simulink model "Battery_Model"  (R2019b)
settings: configuration reference "BMS_Sw_CodeGenConfig" (kept outside this file)
undefined symbols (not defined in the file): Battery, TempInit, ts
libraries: fl_lib x2765, nesl_utility x1565, ee_lib x384, simulink x384, BatteryPack_lib x3
(part 23 of 33)

== system Battery_Model/Battery_Pack/Battery_Pack_7Modules/Cell_3p05/Cell_Module_1 ==
  AmbientTemp : Inport
  Battery_Cell001 : ee_lib/Sources/Battery (Table-Based)  SOC_vec=Battery.SOC_LUT  T_dependence=ee.enum.temperature_dependence.yes  T_vec=Battery.Temperature_LUT K  V0_mat=Battery.Em_LUT V  V0_vec=[3.1, 3.27, 3.31, 3.5] V  R0_mat=Battery.R0_LUT Ohm  R0_vec=[.015, .017, .012, .013] Ohm  AH_vec=Battery.Capacity_LUT hr*A  AH=4.1 hr*A  prm_leak=ee.enum.battery.prm_leak.disabled  Rleak_vec=[8000, 7000, 6000] Ohm  Rleak=7e3 Ohm  prm_dyn=ee.enum.battery.prm_dyn.rc1  R1_mat=Battery.R1_LUT Ohm  R1_vec=[.076, .022, .007, .043] Ohm  tau1_mat=Battery.R1_LUT.*Battery.C1_LUT s  tau1_vec=[148, 110, 27, 22] s  R2_mat=[.014, .382, .407; .028, .006, .007; .014, .007, .006; .333, .956, .912] Ohm  R2_vec=[.382, .006, .007, .956] Ohm  tau2_mat=[1, 44, 5644; 11, 24, 506; 2, 14, 330; 3310, 13419, 30216] s  tau2_vec=[44, 24, 14, 13419] s  R3_mat=[.014, .382, .407; .028, .006, .007; .014, .007, .006; .333, .956, .912] Ohm  R3_vec=[.382, .006, .007, .956] Ohm  tau3_mat=[1, 44, 5644; 11, 24, 506; 2, 14, 330; 3310, 13419, 30216] s  tau3_vec=[44, 24, 14, 13419] s  R4_mat=[.014, .382, .407; .028, .006, .007; .014, .007, .006; .333, .956, .912] Ohm  R4_vec=[.382, .006, .007, .956] Ohm  tau4_mat=[1, 44, 5644; 11, 24, 506; 2, 14, 330; 3310, 13419, 30216] s  tau4_vec=[44, 24, 14, 13419] s  R5_mat=[.014, .382, .407; .028, .006, .007; .014, .007, .006; .333, .956, .912] Ohm  R5_vec=[.382, .006, .007, .956] Ohm  tau5_mat=[1, 44, 5644; 11, 24, 506; 2, 14, 330; 3310, 13419, 30216] s  tau5_vec=[44, 24, 14, 13419] s  prm_fade=ee.enum.battery.prm_fade.equations  N0=100  dV0=0  dR0=0  dAH=0  dRleak=0  dR1=0  dR2=0  dR3=0  dR4=0  dR5=0  N0vec=[100, 200, 300]  Tfadevec=[298.15, 323.15] K  dV0vec=[0, 0, 0]  dR0vec=[0, 0, 0]  dAHvec=[0, 0, 0]  dRleakvec=[0, 0, 0]  dR1vec=[0, 0, 0]  dR2vec=[0, 0, 0]  dR3vec=[0, 0, 0]  dR4vec=[0, 0, 0]  dR5vec=[0, 0, 0]  dV0mat=[0, 0; 0, 0; 0, 0]  dR0mat=[0, 0; 0, 0; 0, 0]  dAHmat=[0, 0; 0, 0; 0, 0]  dRleakmat=[0, 0; 0, 0; 0, 0]  dR1mat=[0, 0; 0, 0; 0, 0]  dR2mat=[0, 0; 0, 0; 0, 0]  dR3mat=[0, 0; 0, 0; 0, 0]  dR4mat=[0, 0; 0, 0; 0, 0]  dR5mat=[0, 0; 0, 0; 0, 0]  temperature=Battery.TempInit K  i_specify=off  i_priority=None  i=0 A  i_nominal_specify=off  i_nominal_unit=A  i_nominal_value=1  v_specify=off  v_priority=None  v=0 V  v_nominal_specify=off  v_nominal_unit=V  v_nominal_value=1  stateOfCharge_specify=on  stateOfCharge_priority=High  stateOfCharge=(Battery.Capacity_LUT(1) - Battery.Qe_init)/Battery.Capacity_LUT(1)  stateOfCharge_nominal_specify=off  stateOfCharge_nominal_unit=1  stateOfCharge_nominal_value=1  num_cycles_specify=off  num_cycles_priority=High  num_cycles=0  num_cycles_nominal_specify=off  num_cycles_nominal_unit=1  num_cycles_nominal_value=1  thermal_mass=Battery.cell_mass*Battery.cell_Cp_heat J/K  temperature_specify=on  temperature_priority=High  temperature_nominal_specify=off  temperature_nominal_unit=K  temperature_nominal_value=1
      settings: SourceProductName=Simscape Electrical  SourceProductBaseCode=PS  InternalSimscapePortConfiguration="{\"Bottom\":[],\"Left\":[{\"id\":\"p\",\"label\":\"+\",\"type\":\"foundation.electrical.electrical\"},{\"id\":\"soc\",\"label\":\"SOC\",\"type\":\"output\"}],\"Right\":[{\"id\":\"n\",\"label\":\"-\",\"type\":\"foundation.electrical.electrical\"},{\"id\":\"H\",\"label\":\"H\",\"type\":\"foundation.thermal.thermal\"}],\"Top\":[]}"
  Battery_Cell002 : ee_lib/Sources/Battery (Table-Based)  SOC_vec=Battery.SOC_LUT  T_dependence=ee.enum.temperature_dependence.yes  T_vec=Battery.Temperature_LUT K  V0_mat=Battery.Em_LUT V  V0_vec=[3.1, 3.27, 3.31, 3.5] V  R0_mat=Battery.R0_LUT Ohm  R0_vec=[.015, .017, .012, .013] Ohm  AH_vec=Battery.Capacity_LUT hr*A  AH=4.1 hr*A  prm_leak=ee.enum.battery.prm_leak.disabled  Rleak_vec=[8000, 7000, 6000] Ohm  Rleak=7e3 Ohm  prm_dyn=ee.enum.battery.prm_dyn.rc1  R1_mat=Battery.R1_LUT Ohm  R1_vec=[.076, .022, .007, .043] Ohm  tau1_mat=Battery.R1_LUT.*Battery.C1_LUT s  tau1_vec=[148, 110, 27, 22] s  R2_mat=[.014, .382, .407; .028, .006, .007; .014, .007, .006; .333, .956, .912] Ohm  R2_vec=[.382, .006, .007, .956] Ohm  tau2_mat=[1, 44, 5644; 11, 24, 506; 2, 14, 330; 3310, 13419, 30216] s  tau2_vec=[44, 24, 14, 13419] s  R3_mat=[.014, .382, .407; .028, .006, .007; .014, .007, .006; .333, .956, .912] Ohm  R3_vec=[.382, .006, .007, .956] Ohm  tau3_mat=[1, 44, 5644; 11, 24, 506; 2, 14, 330; 3310, 13419, 30216] s  tau3_vec=[44, 24, 14, 13419] s  R4_mat=[.014, .382, .407; .028, .006, .007; .014, .007, .006; .333, .956, .912] Ohm  R4_vec=[.382, .006, .007, .956] Ohm  tau4_mat=[1, 44, 5644; 11, 24, 506; 2, 14, 330; 3310, 13419, 30216] s  tau4_vec=[44, 24, 14, 13419] s  R5_mat=[.014, .382, .407; .028, .006, .007; .014, .007, .006; .333, .956, .912] Ohm  R5_vec=[.382, .006, .007, .956] Ohm  tau5_mat=[1, 44, 5644; 11, 24, 506; 2, 14, 330; 3310, 13419, 30216] s  tau5_vec=[44, 24, 14, 13419] s  prm_fade=ee.enum.battery.prm_fade.equations  N0=100  dV0=0  dR0=0  dAH=0  dRleak=0  dR1=0  dR2=0  dR3=0  dR4=0  dR5=0  N0vec=[100, 200, 300]  Tfadevec=[298.15, 323.15] K  dV0vec=[0, 0, 0]  dR0vec=[0, 0, 0]  dAHvec=[0, 0, 0]  dRleakvec=[0, 0, 0]  dR1vec=[0, 0, 0]  dR2vec=[0, 0, 0]  dR3vec=[0, 0, 0]  dR4vec=[0, 0, 0]  dR5vec=[0, 0, 0]  dV0mat=[0, 0; 0, 0; 0, 0]  dR0mat=[0, 0; 0, 0; 0, 0]  dAHmat=[0, 0; 0, 0; 0, 0]  dRleakmat=[0, 0; 0, 0; 0, 0]  dR1mat=[0, 0; 0, 0; 0, 0]  dR2mat=[0, 0; 0, 0; 0, 0]  dR3mat=[0, 0; 0, 0; 0, 0]  dR4mat=[0, 0; 0, 0; 0, 0]  dR5mat=[0, 0; 0, 0; 0, 0]  temperature=Battery.TempInit K  i_specify=off  i_priority=None  i=0 A  i_nominal_specify=off  i_nominal_unit=A  i_nominal_value=1  v_specify=off  v_priority=None  v=0 V  v_nominal_specify=off  v_nominal_unit=V  v_nominal_value=1  stateOfCharge_specify=on  stateOfCharge_priority=High  stateOfCharge=(Battery.Capacity_LUT(1) - Battery.Qe_init)/Battery.Capacity_LUT(1)  stateOfCharge_nominal_specify=off  stateOfCharge_nominal_unit=1  stateOfCharge_nominal_value=1  num_cycles_specify=off  num_cycles_priority=High  num_cycles=0  num_cycles_nominal_specify=off  num_cycles_nominal_unit=1  num_cycles_nominal_value=1  thermal_mass=Battery.cell_mass*Battery.cell_Cp_heat J/K  temperature_specify=on  temperature_priority=High  temperature_nominal_specify=off  temperature_nominal_unit=K  temperature_nominal_value=1
      settings: SourceProductName=Simscape Electrical  SourceProductBaseCode=PS  InternalSimscapePortConfiguration="{\"Bottom\":[],\"Left\":[{\"id\":\"p\",\"label\":\"+\",\"type\":\"foundation.electrical.electrical\"},{\"id\":\"soc\",\"label\":\"SOC\",\"type\":\"output\"}],\"Right\":[{\"id\":\"n\",\"label\":\"-\",\"type\":\"foundation.electrical.electrical\"},{\"id\":\"H\",\"label\":\"H\",\"type\":\"foundation.thermal.thermal\"}],\"Top\":[]}"
  Battery_Cell003 : ee_lib/Sources/Battery (Table-Based)  SOC_vec=Battery.SOC_LUT  T_dependence=ee.enum.temperature_dependence.yes  T_vec=Battery.Temperature_LUT K  V0_mat=Battery.Em_LUT V  V0_vec=[3.1, 3.27, 3.31, 3.5] V  R0_mat=Battery.R0_LUT Ohm  R0_vec=[.015, .017, .012, .013] Ohm  AH_vec=Battery.Capacity_LUT hr*A  AH=4.1 hr*A  prm_leak=ee.enum.battery.prm_leak.disabled  Rleak_vec=[8000, 7000, 6000] Ohm  Rleak=7e3 Ohm  prm_dyn=ee.enum.battery.prm_dyn.rc1  R1_mat=Battery.R1_LUT Ohm  R1_vec=[.076, .022, .007, .043] Ohm  tau1_mat=Battery.R1_LUT.*Battery.C1_LUT s  tau1_vec=[148, 110, 27, 22] s  R2_mat=[.014, .382, .407; .028, .006, .007; .014, .007, .006; .333, .956, .912] Ohm  R2_vec=[.382, .006, .007, .956] Ohm  tau2_mat=[1, 44, 5644; 11, 24, 506; 2, 14, 330; 3310, 13419, 30216] s  tau2_vec=[44, 24, 14, 13419] s  R3_mat=[.014, .382, .407; .028, .006, .007; .014, .007, .006; .333, .956, .912] Ohm  R3_vec=[.382, .006, .007, .956] Ohm  tau3_mat=[1, 44, 5644; 11, 24, 506; 2, 14, 330; 3310, 13419, 30216] s  tau3_vec=[44, 24, 14, 13419] s  R4_mat=[.014, .382, .407; .028, .006, .007; .014, .007, .006; .333, .956, .912] Ohm  R4_vec=[.382, .006, .007, .956] Ohm  tau4_mat=[1, 44, 5644; 11, 24, 506; 2, 14, 330; 3310, 13419, 30216] s  tau4_vec=[44, 24, 14, 13419] s  R5_mat=[.014, .382, .407; .028, .006, .007; .014, .007, .006; .333, .956, .912] Ohm  R5_vec=[.382, .006, .007, .956] Ohm  tau5_mat=[1, 44, 5644; 11, 24, 506; 2, 14, 330; 3310, 13419, 30216] s  tau5_vec=[44, 24, 14, 13419] s  prm_fade=ee.enum.battery.prm_fade.equations  N0=100  dV0=0  dR0=0  dAH=0  dRleak=0  dR1=0  dR2=0  dR3=0  dR4=0  dR5=0  N0vec=[100, 200, 300]  Tfadevec=[298.15, 323.15] K  dV0vec=[0, 0, 0]  dR0vec=[0, 0, 0]  dAHvec=[0, 0, 0]  dRleakvec=[0, 0, 0]  dR1vec=[0, 0, 0]  dR2vec=[0, 0, 0]  dR3vec=[0, 0, 0]  dR4vec=[0, 0, 0]  dR5vec=[0, 0, 0]  dV0mat=[0, 0; 0, 0; 0, 0]  dR0mat=[0, 0; 0, 0; 0, 0]  dAHmat=[0, 0; 0, 0; 0, 0]  dRleakmat=[0, 0; 0, 0; 0, 0]  dR1mat=[0, 0; 0, 0; 0, 0]  dR2mat=[0, 0; 0, 0; 0, 0]  dR3mat=[0, 0; 0, 0; 0, 0]  dR4mat=[0, 0; 0, 0; 0, 0]  dR5mat=[0, 0; 0, 0; 0, 0]  temperature=Battery.TempInit K  i_specify=off  i_priority=None  i=0 A  i_nominal_specify=off  i_nominal_unit=A  i_nominal_value=1  v_specify=off  v_priority=None  v=0 V  v_nominal_specify=off  v_nominal_unit=V  v_nominal_value=1  stateOfCharge_specify=on  stateOfCharge_priority=High  stateOfCharge=(Battery.Capacity_LUT(1) - Battery.Qe_init)/Battery.Capacity_LUT(1)  stateOfCharge_nominal_specify=off  stateOfCharge_nominal_unit=1  stateOfCharge_nominal_value=1  num_cycles_specify=off  num_cycles_priority=High  num_cycles=0  num_cycles_nominal_specify=off  num_cycles_nominal_unit=1  num_cycles_nominal_value=1  thermal_mass=Battery.cell_mass*Battery.cell_Cp_heat J/K  temperature_specify=on  temperature_priority=High  temperature_nominal_specify=off  temperature_nominal_unit=K  temperature_nominal_value=1
      settings: SourceProductName=Simscape Electrical  SourceProductBaseCode=PS  InternalSimscapePortConfiguration="{\"Bottom\":[],\"Left\":[{\"id\":\"p\",\"label\":\"+\",\"type\":\"foundation.electrical.electrical\"},{\"id\":\"soc\",\"label\":\"SOC\",\"type\":\"output\"}],\"Right\":[{\"id\":\"n\",\"label\":\"-\",\"type\":\"foundation.electrical.electrical\"},{\"id\":\"H\",\"label\":\"H\",\"type\":\"foundation.thermal.thermal\"}],\"Top\":[]}"
  Battery_Cell004 : ee_lib/Sources/Battery (Table-Based)  SOC_vec=Battery.SOC_LUT  T_dependence=ee.enum.temperature_dependence.yes  T_vec=Battery.Temperature_LUT K  V0_mat=Battery.Em_LUT V  V0_vec=[3.1, 3.27, 3.31, 3.5] V  R0_mat=Battery.R0_LUT Ohm  R0_vec=[.015, .017, .012, .013] Ohm  AH_vec=Battery.Capacity_LUT hr*A  AH=4.1 hr*A  prm_leak=ee.enum.battery.prm_leak.disabled  Rleak_vec=[8000, 7000, 6000] Ohm  Rleak=7e3 Ohm  prm_dyn=ee.enum.battery.prm_dyn.rc1  R1_mat=Battery.R1_LUT Ohm  R1_vec=[.076, .022, .007, .043] Ohm  tau1_mat=Battery.R1_LUT.*Battery.C1_LUT s  tau1_vec=[148, 110, 27, 22] s  R2_mat=[.014, .382, .407; .028, .006, .007; .014, .007, .006; .333, .956, .912] Ohm  R2_vec=[.382, .006, .007, .956] Ohm  tau2_mat=[1, 44, 5644; 11, 24, 506; 2, 14, 330; 3310, 13419, 30216] s  tau2_vec=[44, 24, 14, 13419] s  R3_mat=[.014, .382, .407; .028, .006, .007; .014, .007, .006; .333, .956, .912] Ohm  R3_vec=[.382, .006, .007, .956] Ohm  tau3_mat=[1, 44, 5644; 11, 24, 506; 2, 14, 330; 3310, 13419, 30216] s  tau3_vec=[44, 24, 14, 13419] s  R4_mat=[.014, .382, .407; .028, .006, .007; .014, .007, .006; .333, .956, .912] Ohm  R4_vec=[.382, .006, .007, .956] Ohm  tau4_mat=[1, 44, 5644; 11, 24, 506; 2, 14, 330; 3310, 13419, 30216] s  tau4_vec=[44, 24, 14, 13419] s  R5_mat=[.014, .382, .407; .028, .006, .007; .014, .007, .006; .333, .956, .912] Ohm  R5_vec=[.382, .006, .007, .956] Ohm  tau5_mat=[1, 44, 5644; 11, 24, 506; 2, 14, 330; 3310, 13419, 30216] s  tau5_vec=[44, 24, 14, 13419] s  prm_fade=ee.enum.battery.prm_fade.equations  N0=100  dV0=0  dR0=0  dAH=0  dRleak=0  dR1=0  dR2=0  dR3=0  dR4=0  dR5=0  N0vec=[100, 200, 300]  Tfadevec=[298.15, 323.15] K  dV0vec=[0, 0, 0]  dR0vec=[0, 0, 0]  dAHvec=[0, 0, 0]  dRleakvec=[0, 0, 0]  dR1vec=[0, 0, 0]  dR2vec=[0, 0, 0]  dR3vec=[0, 0, 0]  dR4vec=[0, 0, 0]  dR5vec=[0, 0, 0]  dV0mat=[0, 0; 0, 0; 0, 0]  dR0mat=[0, 0; 0, 0; 0, 0]  dAHmat=[0, 0; 0, 0; 0, 0]  dRleakmat=[0, 0; 0, 0; 0, 0]  dR1mat=[0, 0; 0, 0; 0, 0]  dR2mat=[0, 0; 0, 0; 0, 0]  dR3mat=[0, 0; 0, 0; 0, 0]  dR4mat=[0, 0; 0, 0; 0, 0]  dR5mat=[0, 0; 0, 0; 0, 0]  temperature=Battery.TempInit K  i_specify=off  i_priority=None  i=0 A  i_nominal_specify=off  i_nominal_unit=A  i_nominal_value=1  v_specify=off  v_priority=None  v=0 V  v_nominal_specify=off  v_nominal_unit=V  v_nominal_value=1  stateOfCharge_specify=on  stateOfCharge_priority=High  stateOfCharge=(Battery.Capacity_LUT(1) - Battery.Qe_init)/Battery.Capacity_LUT(1)  stateOfCharge_nominal_specify=off  stateOfCharge_nominal_unit=1  stateOfCharge_nominal_value=1  num_cycles_specify=off  num_cycles_priority=High  num_cycles=0  num_cycles_nominal_specify=off  num_cycles_nominal_unit=1  num_cycles_nominal_value=1  thermal_mass=Battery.cell_mass*Battery.cell_Cp_heat J/K  temperature_specify=on  temperature_priority=High  temperature_nominal_specify=off  temperature_nominal_unit=K  temperature_nominal_value=1
      settings: SourceProductName=Simscape Electrical  SourceProductBaseCode=PS  InternalSimscapePortConfiguration="{\"Bottom\":[],\"Left\":[{\"id\":\"p\",\"label\":\"+\",\"type\":\"foundation.electrical.electrical\"},{\"id\":\"soc\",\"label\":\"SOC\",\"type\":\"output\"}],\"Right\":[{\"id\":\"n\",\"label\":\"-\",\"type\":\"foundation.electrical.electrical\"},{\"id\":\"H\",\"label\":\"H\",\"type\":\"foundation.thermal.thermal\"}],\"Top\":[]}"
  Battery_Cell005 : ee_lib/Sources/Battery (Table-Based)  SOC_vec=Battery.SOC_LUT  T_dependence=ee.enum.temperature_dependence.yes  T_vec=Battery.Temperature_LUT K  V0_mat=Battery.Em_LUT V  V0_vec=[3.1, 3.27, 3.31, 3.5] V  R0_mat=Battery.R0_LUT Ohm  R0_vec=[.015, .017, .012, .013] Ohm  AH_vec=Battery.Capacity_LUT hr*A  AH=4.1 hr*A  prm_leak=ee.enum.battery.prm_leak.disabled  Rleak_vec=[8000, 7000, 6000] Ohm  Rleak=7e3 Ohm  prm_dyn=ee.enum.battery.prm_dyn.rc1  R1_mat=Battery.R1_LUT Ohm  R1_vec=[.076, .022, .007, .043] Ohm  tau1_mat=Battery.R1_LUT.*Battery.C1_LUT s  tau1_vec=[148, 110, 27, 22] s  R2_mat=[.014, .382, .407; .028, .006, .007; .014, .007, .006; .333, .956, .912] Ohm  R2_vec=[.382, .006, .007, .956] Ohm  tau2_mat=[1, 44, 5644; 11, 24, 506; 2, 14, 330; 3310, 13419, 30216] s  tau2_vec=[44, 24, 14, 13419] s  R3_mat=[.014, .382, .407; .028, .006, .007; .014, .007, .006; .333, .956, .912] Ohm  R3_vec=[.382, .006, .007, .956] Ohm  tau3_mat=[1, 44, 5644; 11, 24, 506; 2, 14, 330; 3310, 13419, 30216] s  tau3_vec=[44, 24, 14, 13419] s  R4_mat=[.014, .382, .407; .028, .006, .007; .014, .007, .006; .333, .956, .912] Ohm  R4_vec=[.382, .006, .007, .956] Ohm  tau4_mat=[1, 44, 5644; 11, 24, 506; 2, 14, 330; 3310, 13419, 30216] s  tau4_vec=[44, 24, 14, 13419] s  R5_mat=[.014, .382, .407; .028, .006, .007; .014, .007, .006; .333, .956, .912] Ohm  R5_vec=[.382, .006, .007, .956] Ohm  tau5_mat=[1, 44, 5644; 11, 24, 506; 2, 14, 330; 3310, 13419, 30216] s  tau5_vec=[44, 24, 14, 13419] s  prm_fade=ee.enum.battery.prm_fade.equations  N0=100  dV0=0  dR0=0  dAH=0  dRleak=0  dR1=0  dR2=0  dR3=0  dR4=0  dR5=0  N0vec=[100, 200, 300]  Tfadevec=[298.15, 323.15] K  dV0vec=[0, 0, 0]  dR0vec=[0, 0, 0]  dAHvec=[0, 0, 0]  dRleakvec=[0, 0, 0]  dR1vec=[0, 0, 0]  dR2vec=[0, 0, 0]  dR3vec=[0, 0, 0]  dR4vec=[0, 0, 0]  dR5vec=[0, 0, 0]  dV0mat=[0, 0; 0, 0; 0, 0]  dR0mat=[0, 0; 0, 0; 0, 0]  dAHmat=[0, 0; 0, 0; 0, 0]  dRleakmat=[0, 0; 0, 0; 0, 0]  dR1mat=[0, 0; 0, 0; 0, 0]  dR2mat=[0, 0; 0, 0; 0, 0]  dR3mat=[0, 0; 0, 0; 0, 0]  dR4mat=[0, 0; 0, 0; 0, 0]  dR5mat=[0, 0; 0, 0; 0, 0]  temperature=Battery.TempInit K  i_specify=off  i_priority=None  i=0 A  i_nominal_specify=off  i_nominal_unit=A  i_nominal_value=1  v_specify=off  v_priority=None  v=0 V  v_nominal_specify=off  v_nominal_unit=V  v_nominal_value=1  stateOfCharge_specify=on  stateOfCharge_priority=High  stateOfCharge=(Battery.Capacity_LUT(1) - Battery.Qe_init)/Battery.Capacity_LUT(1)  stateOfCharge_nominal_specify=off  stateOfCharge_nominal_unit=1  stateOfCharge_nominal_value=1  num_cycles_specify=off  num_cycles_priority=High  num_cycles=0  num_cycles_nominal_specify=off  num_cycles_nominal_unit=1  num_cycles_nominal_value=1  thermal_mass=Battery.cell_mass*Battery.cell_Cp_heat J/K  temperature_specify=on  temperature_priority=High  temperature_nominal_specify=off  temperature_nominal_unit=K  temperature_nominal_value=1
      settings: SourceProductName=Simscape Electrical  SourceProductBaseCode=PS  InternalSimscapePortConfiguration="{\"Bottom\":[],\"Left\":[{\"id\":\"p\",\"label\":\"+\",\"type\":\"foundation.electrical.electrical\"},{\"id\":\"soc\",\"label\":\"SOC\",\"type\":\"output\"}],\"Right\":[{\"id\":\"n\",\"label\":\"-\",\"type\":\"foundation.electrical.electrical\"},{\"id\":\"H\",\"label\":\"H\",\"type\":\"foundation.thermal.thermal\"}],\"Top\":[]}"
  Battery_Cell006 : ee_lib/Sources/Battery (Table-Based)  SOC_vec=Battery.SOC_LUT  T_dependence=ee.enum.temperature_dependence.yes  T_vec=Battery.Temperature_LUT K  V0_mat=Battery.Em_LUT V  V0_vec=[3.1, 3.27, 3.31, 3.5] V  R0_mat=Battery.R0_LUT Ohm  R0_vec=[.015, .017, .012, .013] Ohm  AH_vec=Battery.Capacity_LUT hr*A  AH=4.1 hr*A  prm_leak=ee.enum.battery.prm_leak.disabled  Rleak_vec=[8000, 7000, 6000] Ohm  Rleak=7e3 Ohm  prm_dyn=ee.enum.battery.prm_dyn.rc1  R1_mat=Battery.R1_LUT Ohm  R1_vec=[.076, .022, .007, .043] Ohm  tau1_mat=Battery.R1_LUT.*Battery.C1_LUT s  tau1_vec=[148, 110, 27, 22] s  R2_mat=[.014, .382, .407; .028, .006, .007; .014, .007, .006; .333, .956, .912] Ohm  R2_vec=[.382, .006, .007, .956] Ohm  tau2_mat=[1, 44, 5644; 11, 24, 506; 2, 14, 330; 3310, 13419, 30216] s  tau2_vec=[44, 24, 14, 13419] s  R3_mat=[.014, .382, .407; .028, .006, .007; .014, .007, .006; .333, .956, .912] Ohm  R3_vec=[.382, .006, .007, .956] Ohm  tau3_mat=[1, 44, 5644; 11, 24, 506; 2, 14, 330; 3310, 13419, 30216] s  tau3_vec=[44, 24, 14, 13419] s  R4_mat=[.014, .382, .407; .028, .006, .007; .014, .007, .006; .333, .956, .912] Ohm  R4_vec=[.382, .006, .007, .956] Ohm  tau4_mat=[1, 44, 5644; 11, 24, 506; 2, 14, 330; 3310, 13419, 30216] s  tau4_vec=[44, 24, 14, 13419] s  R5_mat=[.014, .382, .407; .028, .006, .007; .014, .007, .006; .333, .956, .912] Ohm  R5_vec=[.382, .006, .007, .956] Ohm  tau5_mat=[1, 44, 5644; 11, 24, 506; 2, 14, 330; 3310, 13419, 30216] s  tau5_vec=[44, 24, 14, 13419] s  prm_fade=ee.enum.battery.prm_fade.equations  N0=100  dV0=0  dR0=0  dAH=0  dRleak=0  dR1=0  dR2=0  dR3=0  dR4=0  dR5=0  N0vec=[100, 200, 300]  Tfadevec=[298.15, 323.15] K  dV0vec=[0, 0, 0]  dR0vec=[0, 0, 0]  dAHvec=[0, 0, 0]  dRleakvec=[0, 0, 0]  dR1vec=[0, 0, 0]  dR2vec=[0, 0, 0]  dR3vec=[0, 0, 0]  dR4vec=[0, 0, 0]  dR5vec=[0, 0, 0]  dV0mat=[0, 0; 0, 0; 0, 0]  dR0mat=[0, 0; 0, 0; 0, 0]  dAHmat=[0, 0; 0, 0; 0, 0]  dRleakmat=[0, 0; 0, 0; 0, 0]  dR1mat=[0, 0; 0, 0; 0, 0]  dR2mat=[0, 0; 0, 0; 0, 0]  dR3mat=[0, 0; 0, 0; 0, 0]  dR4mat=[0, 0; 0, 0; 0, 0]  dR5mat=[0, 0; 0, 0; 0, 0]  temperature=Battery.TempInit K  i_specify=off  i_priority=None  i=0 A  i_nominal_specify=off  i_nominal_unit=A  i_nominal_value=1  v_specify=off  v_priority=None  v=0 V  v_nominal_specify=off  v_nominal_unit=V  v_nominal_value=1  stateOfCharge_specify=on  stateOfCharge_priority=High  stateOfCharge=(Battery.Capacity_LUT(1) - Battery.Qe_init)/Battery.Capacity_LUT(1)  stateOfCharge_nominal_specify=off  stateOfCharge_nominal_unit=1  stateOfCharge_nominal_value=1  num_cycles_specify=off  num_cycles_priority=High  num_cycles=0  num_cycles_nominal_specify=off  num_cycles_nominal_unit=1  num_cycles_nominal_value=1  thermal_mass=Battery.cell_mass*Battery.cell_Cp_heat J/K  temperature_specify=on  temperature_priority=High  temperature_nominal_specify=off  temperature_nominal_unit=K  temperature_nominal_value=1
      settings: SourceProductName=Simscape Electrical  SourceProductBaseCode=PS  InternalSimscapePortConfiguration="{\"Bottom\":[],\"Left\":[{\"id\":\"p\",\"label\":\"+\",\"type\":\"foundation.electrical.electrical\"},{\"id\":\"soc\",\"label\":\"SOC\",\"type\":\"output\"}],\"Right\":[{\"id\":\"n\",\"label\":\"-\",\"type\":\"foundation.electrical.electrical\"},{\"id\":\"H\",\"label\":\"H\",\"type\":\"foundation.thermal.thermal\"}],\"Top\":[]}"
  Battery_Cell007 : ee_lib/Sources/Battery (Table-Based)  SOC_vec=Battery.SOC_LUT  T_dependence=ee.enum.temperature_dependence.yes  T_vec=Battery.Temperature_LUT K  V0_mat=Battery.Em_LUT V  V0_vec=[3.1, 3.27, 3.31, 3.5] V  R0_mat=Battery.R0_LUT Ohm  R0_vec=[.015, .017, .012, .013] Ohm  AH_vec=Battery.Capacity_LUT hr*A  AH=4.1 hr*A  prm_leak=ee.enum.battery.prm_leak.disabled  Rleak_vec=[8000, 7000, 6000] Ohm  Rleak=7e3 Ohm  prm_dyn=ee.enum.battery.prm_dyn.rc1  R1_mat=Battery.R1_LUT Ohm  R1_vec=[.076, .022, .007, .043] Ohm  tau1_mat=Battery.R1_LUT.*Battery.C1_LUT s  tau1_vec=[148, 110, 27, 22] s  R2_mat=[.014, .382, .407; .028, .006, .007; .014, .007, .006; .333, .956, .912] Ohm  R2_vec=[.382, .006, .007, .956] Ohm  tau2_mat=[1, 44, 5644; 11, 24, 506; 2, 14, 330; 3310, 13419, 30216] s  tau2_vec=[44, 24, 14, 13419] s  R3_mat=[.014, .382, .407; .028, .006, .007; .014, .007, .006; .333, .956, .912] Ohm  R3_vec=[.382, .006, .007, .956] Ohm  tau3_mat=[1, 44, 5644; 11, 24, 506; 2, 14, 330; 3310, 13419, 30216] s  tau3_vec=[44, 24, 14, 13419] s  R4_mat=[.014, .382, .407; .028, .006, .007; .014, .007, .006; .333, .956, .912] Ohm  R4_vec=[.382, .006, .007, .956] Ohm  tau4_mat=[1, 44, 5644; 11, 24, 506; 2, 14, 330; 3310, 13419, 30216] s  tau4_vec=[44, 24, 14, 13419] s  R5_mat=[.014, .382, .407; .028, .006, .007; .014, .007, .006; .333, .956, .912] Ohm  R5_vec=[.382, .006, .007, .956] Ohm  tau5_mat=[1, 44, 5644; 11, 24, 506; 2, 14, 330; 3310, 13419, 30216] s  tau5_vec=[44, 24, 14, 13419] s  prm_fade=ee.enum.battery.prm_fade.equations  N0=100  dV0=0  dR0=0  dAH=0  dRleak=0  dR1=0  dR2=0  dR3=0  dR4=0  dR5=0  N0vec=[100, 200, 300]  Tfadevec=[298.15, 323.15] K  dV0vec=[0, 0, 0]  dR0vec=[0, 0, 0]  dAHvec=[0, 0, 0]  dRleakvec=[0, 0, 0]  dR1vec=[0, 0, 0]  dR2vec=[0, 0, 0]  dR3vec=[0, 0, 0]  dR4vec=[0, 0, 0]  dR5vec=[0, 0, 0]  dV0mat=[0, 0; 0, 0; 0, 0]  dR0mat=[0, 0; 0, 0; 0, 0]  dAHmat=[0, 0; 0, 0; 0, 0]  dRleakmat=[0, 0; 0, 0; 0, 0]  dR1mat=[0, 0; 0, 0; 0, 0]  dR2mat=[0, 0; 0, 0; 0, 0]  dR3mat=[0, 0; 0, 0; 0, 0]  dR4mat=[0, 0; 0, 0; 0, 0]  dR5mat=[0, 0; 0, 0; 0, 0]  temperature=Battery.TempInit K  i_specify=off  i_priority=None  i=0 A  i_nominal_specify=off  i_nominal_unit=A  i_nominal_value=1  v_specify=off  v_priority=None  v=0 V  v_nominal_specify=off  v_nominal_unit=V  v_nominal_value=1  stateOfCharge_specify=on  stateOfCharge_priority=High  stateOfCharge=(Battery.Capacity_LUT(1) - Battery.Qe_init)/Battery.Capacity_LUT(1)  stateOfCharge_nominal_specify=off  stateOfCharge_nominal_unit=1  stateOfCharge_nominal_value=1  num_cycles_specify=off  num_cycles_priority=High  num_cycles=0  num_cycles_nominal_specify=off  num_cycles_nominal_unit=1  num_cycles_nominal_value=1  thermal_mass=Battery.cell_mass*Battery.cell_Cp_heat J/K  temperature_specify=on  temperature_priority=High  temperature_nominal_specify=off  temperature_nominal_unit=K  temperature_nominal_value=1
      settings: SourceProductName=Simscape Electrical  SourceProductBaseCode=PS  InternalSimscapePortConfiguration="{\"Bottom\":[],\"Left\":[{\"id\":\"p\",\"label\":\"+\",\"type\":\"foundation.electrical.electrical\"},{\"id\":\"soc\",\"label\":\"SOC\",\"type\":\"output\"}],\"Right\":[{\"id\":\"n\",\"label\":\"-\",\"type\":\"foundation.electrical.electrical\"},{\"id\":\"H\",\"label\":\"H\",\"type\":\"foundation.thermal.thermal\"}],\"Top\":[]}"
  Battery_Cell008 : ee_lib/Sources/Battery (Table-Based)  SOC_vec=Battery.SOC_LUT  T_dependence=ee.enum.temperature_dependence.yes  T_vec=Battery.Temperature_LUT K  V0_mat=Battery.Em_LUT V  V0_vec=[3.1, 3.27, 3.31, 3.5] V  R0_mat=Battery.R0_LUT Ohm  R0_vec=[.015, .017, .012, .013] Ohm  AH_vec=Battery.Capacity_LUT hr*A  AH=4.1 hr*A  prm_leak=ee.enum.battery.prm_leak.disabled  Rleak_vec=[8000, 7000, 6000] Ohm  Rleak=7e3 Ohm  prm_dyn=ee.enum.battery.prm_dyn.rc1  R1_mat=Battery.R1_LUT Ohm  R1_vec=[.076, .022, .007, .043] Ohm  tau1_mat=Battery.R1_LUT.*Battery.C1_LUT s  tau1_vec=[148, 110, 27, 22] s  R2_mat=[.014, .382, .407; .028, .006, .007; .014, .007, .006; .333, .956, .912] Ohm  R2_vec=[.382, .006, .007, .956] Ohm  tau2_mat=[1, 44, 5644; 11, 24, 506; 2, 14, 330; 3310, 13419, 30216] s  tau2_vec=[44, 24, 14, 13419] s  R3_mat=[.014, .382, .407; .028, .006, .007; .014, .007, .006; .333, .956, .912] Ohm  R3_vec=[.382, .006, .007, .956] Ohm  tau3_mat=[1, 44, 5644; 11, 24, 506; 2, 14, 330; 3310, 13419, 30216] s  tau3_vec=[44, 24, 14, 13419] s  R4_mat=[.014, .382, .407; .028, .006, .007; .014, .007, .006; .333, .956, .912] Ohm  R4_vec=[.382, .006, .007, .956] Ohm  tau4_mat=[1, 44, 5644; 11, 24, 506; 2, 14, 330; 3310, 13419, 30216] s  tau4_vec=[44, 24, 14, 13419] s  R5_mat=[.014, .382, .407; .028, .006, .007; .014, .007, .006; .333, .956, .912] Ohm  R5_vec=[.382, .006, .007, .956] Ohm  tau5_mat=[1, 44, 5644; 11, 24, 506; 2, 14, 330; 3310, 13419, 30216] s  tau5_vec=[44, 24, 14, 13419] s  prm_fade=ee.enum.battery.prm_fade.equations  N0=100  dV0=0  dR0=0  dAH=0  dRleak=0  dR1=0  dR2=0  dR3=0  dR4=0  dR5=0  N0vec=[100, 200, 300]  Tfadevec=[298.15, 323.15] K  dV0vec=[0, 0, 0]  dR0vec=[0, 0, 0]  dAHvec=[0, 0, 0]  dRleakvec=[0, 0, 0]  dR1vec=[0, 0, 0]  dR2vec=[0, 0, 0]  dR3vec=[0, 0, 0]  dR4vec=[0, 0, 0]  dR5vec=[0, 0, 0]  dV0mat=[0, 0; 0, 0; 0, 0]  dR0mat=[0, 0; 0, 0; 0, 0]  dAHmat=[0, 0; 0, 0; 0, 0]  dRleakmat=[0, 0; 0, 0; 0, 0]  dR1mat=[0, 0; 0, 0; 0, 0]  dR2mat=[0, 0; 0, 0; 0, 0]  dR3mat=[0, 0; 0, 0; 0, 0]  dR4mat=[0, 0; 0, 0; 0, 0]  dR5mat=[0, 0; 0, 0; 0, 0]  temperature=Battery.TempInit K  i_specify=off  i_priority=None  i=0 A  i_nominal_specify=off  i_nominal_unit=A  i_nominal_value=1  v_specify=off  v_priority=None  v=0 V  v_nominal_specify=off  v_nominal_unit=V  v_nominal_value=1  stateOfCharge_specify=on  stateOfCharge_priority=High  stateOfCharge=(Battery.Capacity_LUT(1) - Battery.Qe_init)/Battery.Capacity_LUT(1)  stateOfCharge_nominal_specify=off  stateOfCharge_nominal_unit=1  stateOfCharge_nominal_value=1  num_cycles_specify=off  num_cycles_priority=High  num_cycles=0  num_cycles_nominal_specify=off  num_cycles_nominal_unit=1  num_cycles_nominal_value=1  thermal_mass=Battery.cell_mass*Battery.cell_Cp_heat J/K  temperature_specify=on  temperature_priority=High  temperature_nominal_specify=off  temperature_nominal_unit=K  temperature_nominal_value=1
      settings: SourceProductName=Simscape Electrical  SourceProductBaseCode=PS  InternalSimscapePortConfiguration="{\"Bottom\":[],\"Left\":[{\"id\":\"p\",\"label\":\"+\",\"type\":\"foundation.electrical.electrical\"},{\"id\":\"soc\",\"label\":\"SOC\",\"type\":\"output\"}],\"Right\":[{\"id\":\"n\",\"label\":\"-\",\"type\":\"foundation.electrical.electrical\"},{\"id\":\"H\",\"label\":\"H\",\"type\":\"foundation.thermal.thermal\"}],\"Top\":[]}"
  Battery_Cell009 : ee_lib/Sources/Battery (Table-Based)  SOC_vec=Battery.SOC_LUT  T_dependence=ee.enum.temperature_dependence.yes  T_vec=Battery.Temperature_LUT K  V0_mat=Battery.Em_LUT V  V0_vec=[3.1, 3.27, 3.31, 3.5] V  R0_mat=Battery.R0_LUT Ohm  R0_vec=[.015, .017, .012, .013] Ohm  AH_vec=Battery.Capacity_LUT hr*A  AH=4.1 hr*A  prm_leak=ee.enum.battery.prm_leak.disabled  Rleak_vec=[8000, 7000, 6000] Ohm  Rleak=7e3 Ohm  prm_dyn=ee.enum.battery.prm_dyn.rc1  R1_mat=Battery.R1_LUT Ohm  R1_vec=[.076, .022, .007, .043] Ohm  tau1_mat=Battery.R1_LUT.*Battery.C1_LUT s  tau1_vec=[148, 110, 27, 22] s  R2_mat=[.014, .382, .407; .028, .006, .007; .014, .007, .006; .333, .956, .912] Ohm  R2_vec=[.382, .006, .007, .956] Ohm  tau2_mat=[1, 44, 5644; 11, 24, 506; 2, 14, 330; 3310, 13419, 30216] s  tau2_vec=[44, 24, 14, 13419] s  R3_mat=[.014, .382, .407; .028, .006, .007; .014, .007, .006; .333, .956, .912] Ohm  R3_vec=[.382, .006, .007, .956] Ohm  tau3_mat=[1, 44, 5644; 11, 24, 506; 2, 14, 330; 3310, 13419, 30216] s  tau3_vec=[44, 24, 14, 13419] s  R4_mat=[.014, .382, .407; .028, .006, .007; .014, .007, .006; .333, .956, .912] Ohm  R4_vec=[.382, .006, .007, .956] Ohm  tau4_mat=[1, 44, 5644; 11, 24, 506; 2, 14, 330; 3310, 13419, 30216] s  tau4_vec=[44, 24, 14, 13419] s  R5_mat=[.014, .382, .407; .028, .006, .007; .014, .007, .006; .333, .956, .912] Ohm  R5_vec=[.382, .006, .007, .956] Ohm  tau5_mat=[1, 44, 5644; 11, 24, 506; 2, 14, 330; 3310, 13419, 30216] s  tau5_vec=[44, 24, 14, 13419] s  prm_fade=ee.enum.battery.prm_fade.equations  N0=100  dV0=0  dR0=0  dAH=0  dRleak=0  dR1=0  dR2=0  dR3=0  dR4=0  dR5=0  N0vec=[100, 200, 300]  Tfadevec=[298.15, 323.15] K  dV0vec=[0, 0, 0]  dR0vec=[0, 0, 0]  dAHvec=[0, 0, 0]  dRleakvec=[0, 0, 0]  dR1vec=[0, 0, 0]  dR2vec=[0, 0, 0]  dR3vec=[0, 0, 0]  dR4vec=[0, 0, 0]  dR5vec=[0, 0, 0]  dV0mat=[0, 0; 0, 0; 0, 0]  dR0mat=[0, 0; 0, 0; 0, 0]  dAHmat=[0, 0; 0, 0; 0, 0]  dRleakmat=[0, 0; 0, 0; 0, 0]  dR1mat=[0, 0; 0, 0; 0, 0]  dR2mat=[0, 0; 0, 0; 0, 0]  dR3mat=[0, 0; 0, 0; 0, 0]  dR4mat=[0, 0; 0, 0; 0, 0]  dR5mat=[0, 0; 0, 0; 0, 0]  temperature=Battery.TempInit K  i_specify=off  i_priority=None  i=0 A  i_nominal_specify=off  i_nominal_unit=A  i_nominal_value=1  v_specify=off  v_priority=None  v=0 V  v_nominal_specify=off  v_nominal_unit=V  v_nominal_value=1  stateOfCharge_specify=on  stateOfCharge_priority=High  stateOfCharge=(Battery.Capacity_LUT(1) - Battery.Qe_init)/Battery.Capacity_LUT(1)  stateOfCharge_nominal_specify=off  stateOfCharge_nominal_unit=1  stateOfCharge_nominal_value=1  num_cycles_specify=off  num_cycles_priority=High  num_cycles=0  num_cycles_nominal_specify=off  num_cycles_nominal_unit=1  num_cycles_nominal_value=1  thermal_mass=Battery.cell_mass*Battery.cell_Cp_heat J/K  temperature_specify=on  temperature_priority=High  temperature_nominal_specify=off  temperature_nominal_unit=K  temperature_nominal_value=1
      settings: SourceProductName=Simscape Electrical  SourceProductBaseCode=PS  InternalSimscapePortConfiguration="{\"Bottom\":[],\"Left\":[{\"id\":\"p\",\"label\":\"+\",\"type\":\"foundation.electrical.electrical\"},{\"id\":\"soc\",\"label\":\"SOC\",\"type\":\"output\"}],\"Right\":[{\"id\":\"n\",\"label\":\"-\",\"type\":\"foundation.electrical.electrical\"},{\"id\":\"H\",\"label\":\"H\",\"type\":\"foundation.thermal.thermal\"}],\"Top\":[]}"
  Battery_Cell010 : ee_lib/Sources/Battery (Table-Based)  SOC_vec=Battery.SOC_LUT  T_dependence=ee.enum.temperature_dependence.yes  T_vec=Battery.Temperature_LUT K  V0_mat=Battery.Em_LUT V  V0_vec=[3.1, 3.27, 3.31, 3.5] V  R0_mat=Battery.R0_LUT Ohm  R0_vec=[.015, .017, .012, .013] Ohm  AH_vec=Battery.Capacity_LUT hr*A  AH=4.1 hr*A  prm_leak=ee.enum.battery.prm_leak.disabled  Rleak_vec=[8000, 7000, 6000] Ohm  Rleak=7e3 Ohm  prm_dyn=ee.enum.battery.prm_dyn.rc1  R1_mat=Battery.R1_LUT Ohm  R1_vec=[.076, .022, .007, .043] Ohm  tau1_mat=Battery.R1_LUT.*Battery.C1_LUT s  tau1_vec=[148, 110, 27, 22] s  R2_mat=[.014, .382, .407; .028, .006, .007; .014, .007, .006; .333, .956, .912] Ohm  R2_vec=[.382, .006, .007, .956] Ohm  tau2_mat=[1, 44, 5644; 11, 24, 506; 2, 14, 330; 3310, 13419, 30216] s  tau2_vec=[44, 24, 14, 13419] s  R3_mat=[.014, .382, .407; .028, .006, .007; .014, .007, .006; .333, .956, .912] Ohm  R3_vec=[.382, .006, .007, .956] Ohm  tau3_mat=[1, 44, 5644; 11, 24, 506; 2, 14, 330; 3310, 13419, 30216] s  tau3_vec=[44, 24, 14, 13419] s  R4_mat=[.014, .382, .407; .028, .006, .007; .014, .007, .006; .333, .956, .912] Ohm  R4_vec=[.382, .006, .007, .956] Ohm  tau4_mat=[1, 44, 5644; 11, 24, 506; 2, 14, 330; 3310, 13419, 30216] s  tau4_vec=[44, 24, 14, 13419] s  R5_mat=[.014, .382, .407; .028, .006, .007; .014, .007, .006; .333, .956, .912] Ohm  R5_vec=[.382, .006, .007, .956] Ohm  tau5_mat=[1, 44, 5644; 11, 24, 506; 2, 14, 330; 3310, 13419, 30216] s  tau5_vec=[44, 24, 14, 13419] s  prm_fade=ee.enum.battery.prm_fade.equations  N0=100  dV0=0  dR0=0  dAH=0  dRleak=0  dR1=0  dR2=0  dR3=0  dR4=0  dR5=0  N0vec=[100, 200, 300]  Tfadevec=[298.15, 323.15] K  dV0vec=[0, 0, 0]  dR0vec=[0, 0, 0]  dAHvec=[0, 0, 0]  dRleakvec=[0, 0, 0]  dR1vec=[0, 0, 0]  dR2vec=[0, 0, 0]  dR3vec=[0, 0, 0]  dR4vec=[0, 0, 0]  dR5vec=[0, 0, 0]  dV0mat=[0, 0; 0, 0; 0, 0]  dR0mat=[0, 0; 0, 0; 0, 0]  dAHmat=[0, 0; 0, 0; 0, 0]  dRleakmat=[0, 0; 0, 0; 0, 0]  dR1mat=[0, 0; 0, 0; 0, 0]  dR2mat=[0, 0; 0, 0; 0, 0]  dR3mat=[0, 0; 0, 0; 0, 0]  dR4mat=[0, 0; 0, 0; 0, 0]  dR5mat=[0, 0; 0, 0; 0, 0]  temperature=Battery.TempInit K  i_specify=off  i_priority=None  i=0 A  i_nominal_specify=off  i_nominal_unit=A  i_nominal_value=1  v_specify=off  v_priority=None  v=0 V  v_nominal_specify=off  v_nominal_unit=V  v_nominal_value=1  stateOfCharge_specify=on  stateOfCharge_priority=High  stateOfCharge=(Battery.Capacity_LUT(1) - Battery.Qe_init)/Battery.Capacity_LUT(1)  stateOfCharge_nominal_specify=off  stateOfCharge_nominal_unit=1  stateOfCharge_nominal_value=1  num_cycles_specify=off  num_cycles_priority=High  num_cycles=0  num_cycles_nominal_specify=off  num_cycles_nominal_unit=1  num_cycles_nominal_value=1  thermal_mass=Battery.cell_mass*Battery.cell_Cp_heat J/K  temperature_specify=on  temperature_priority=High  temperature_nominal_specify=off  temperature_nominal_unit=K  temperature_nominal_value=1
      settings: SourceProductName=Simscape Electrical  SourceProductBaseCode=PS  InternalSimscapePortConfiguration="{\"Bottom\":[],\"Left\":[{\"id\":\"p\",\"label\":\"+\",\"type\":\"foundation.electrical.electrical\"},{\"id\":\"soc\",\"label\":\"SOC\",\"type\":\"output\"}],\"Right\":[{\"id\":\"n\",\"label\":\"-\",\"type\":\"foundation.electrical.electrical\"},{\"id\":\"H\",\"label\":\"H\",\"type\":\"foundation.thermal.thermal\"}],\"Top\":[]}"
  Battery_Cell011 : ee_lib/Sources/Battery (Table-Based)  SOC_vec=Battery.SOC_LUT  T_dependence=ee.enum.temperature_dependence.yes  T_vec=Battery.Temperature_LUT K  V0_mat=Battery.Em_LUT V  V0_vec=[3.1, 3.27, 3.31, 3.5] V  R0_mat=Battery.R0_LUT Ohm  R0_vec=[.015, .017, .012, .013] Ohm  AH_vec=Battery.Capacity_LUT hr*A  AH=4.1 hr*A  prm_leak=ee.enum.battery.prm_leak.disabled  Rleak_vec=[8000, 7000, 6000] Ohm  Rleak=7e3 Ohm  prm_dyn=ee.enum.battery.prm_dyn.rc1  R1_mat=Battery.R1_LUT Ohm  R1_vec=[.076, .022, .007, .043] Ohm  tau1_mat=Battery.R1_LUT.*Battery.C1_LUT s  tau1_vec=[148, 110, 27, 22] s  R2_mat=[.014, .382, .407; .028, .006, .007; .014, .007, .006; .333, .956, .912] Ohm  R2_vec=[.382, .006, .007, .956] Ohm  tau2_mat=[1, 44, 5644; 11, 24, 506; 2, 14, 330; 3310, 13419, 30216] s  tau2_vec=[44, 24, 14, 13419] s  R3_mat=[.014, .382, .407; .028, .006, .007; .014, .007, .006; .333, .956, .912] Ohm  R3_vec=[.382, .006, .007, .956] Ohm  tau3_mat=[1, 44, 5644; 11, 24, 506; 2, 14, 330; 3310, 13419, 30216] s  tau3_vec=[44, 24, 14, 13419] s  R4_mat=[.014, .382, .407; .028, .006, .007; .014, .007, .006; .333, .956, .912] Ohm  R4_vec=[.382, .006, .007, .956] Ohm  tau4_mat=[1, 44, 5644; 11, 24, 506; 2, 14, 330; 3310, 13419, 30216] s  tau4_vec=[44, 24, 14, 13419] s  R5_mat=[.014, .382, .407; .028, .006, .007; .014, .007, .006; .333, .956, .912] Ohm  R5_vec=[.382, .006, .007, .956] Ohm  tau5_mat=[1, 44, 5644; 11, 24, 506; 2, 14, 330; 3310, 13419, 30216] s  tau5_vec=[44, 24, 14, 13419] s  prm_fade=ee.enum.battery.prm_fade.equations  N0=100  dV0=0  dR0=0  dAH=0  dRleak=0  dR1=0  dR2=0  dR3=0  dR4=0  dR5=0  N0vec=[100, 200, 300]  Tfadevec=[298.15, 323.15] K  dV0vec=[0, 0, 0]  dR0vec=[0, 0, 0]  dAHvec=[0, 0, 0]  dRleakvec=[0, 0, 0]  dR1vec=[0, 0, 0]  dR2vec=[0, 0, 0]  dR3vec=[0, 0, 0]  dR4vec=[0, 0, 0]  dR5vec=[0, 0, 0]  dV0mat=[0, 0; 0, 0; 0, 0]  dR0mat=[0, 0; 0, 0; 0, 0]  dAHmat=[0, 0; 0, 0; 0, 0]  dRleakmat=[0, 0; 0, 0; 0, 0]  dR1mat=[0, 0; 0, 0; 0, 0]  dR2mat=[0, 0; 0, 0; 0, 0]  dR3mat=[0, 0; 0, 0; 0, 0]  dR4mat=[0, 0; 0, 0; 0, 0]  dR5mat=[0, 0; 0, 0; 0, 0]  temperature=Battery.TempInit K  i_specify=off  i_priority=None  i=0 A  i_nominal_specify=off  i_nominal_unit=A  i_nominal_value=1  v_specify=off  v_priority=None  v=0 V  v_nominal_specify=off  v_nominal_unit=V  v_nominal_value=1  stateOfCharge_specify=on  stateOfCharge_priority=High  stateOfCharge=(Battery.Capacity_LUT(1) - Battery.Qe_init)/Battery.Capacity_LUT(1)  stateOfCharge_nominal_specify=off  stateOfCharge_nominal_unit=1  stateOfCharge_nominal_value=1  num_cycles_specify=off  num_cycles_priority=High  num_cycles=0  num_cycles_nominal_specify=off  num_cycles_nominal_unit=1  num_cycles_nominal_value=1  thermal_mass=Battery.cell_mass*Battery.cell_Cp_heat J/K  temperature_specify=on  temperature_priority=High  temperature_nominal_specify=off  temperature_nominal_unit=K  temperature_nominal_value=1
      settings: SourceProductName=Simscape Electrical  SourceProductBaseCode=PS  InternalSimscapePortConfiguration="{\"Bottom\":[],\"Left\":[{\"id\":\"p\",\"label\":\"+\",\"type\":\"foundation.electrical.electrical\"},{\"id\":\"soc\",\"label\":\"SOC\",\"type\":\"output\"}],\"Right\":[{\"id\":\"n\",\"label\":\"-\",\"type\":\"foundation.electrical.electrical\"},{\"id\":\"H\",\"label\":\"H\",\"type\":\"foundation.thermal.thermal\"}],\"Top\":[]}"
  Battery_Cell012 : ee_lib/Sources/Battery (Table-Based)  SOC_vec=Battery.SOC_LUT  T_dependence=ee.enum.temperature_dependence.yes  T_vec=Battery.Temperature_LUT K  V0_mat=Battery.Em_LUT V  V0_vec=[3.1, 3.27, 3.31, 3.5] V  R0_mat=Battery.R0_LUT Ohm  R0_vec=[.015, .017, .012, .013] Ohm  AH_vec=Battery.Capacity_LUT hr*A  AH=4.1 hr*A  prm_leak=ee.enum.battery.prm_leak.disabled  Rleak_vec=[8000, 7000, 6000] Ohm  Rleak=7e3 Ohm  prm_dyn=ee.enum.battery.prm_dyn.rc1  R1_mat=Battery.R1_LUT Ohm  R1_vec=[.076, .022, .007, .043] Ohm  tau1_mat=Battery.R1_LUT.*Battery.C1_LUT s  tau1_vec=[148, 110, 27, 22] s  R2_mat=[.014, .382, .407; .028, .006, .007; .014, .007, .006; .333, .956, .912] Ohm  R2_vec=[.382, .006, .007, .956] Ohm  tau2_mat=[1, 44, 5644; 11, 24, 506; 2, 14, 330; 3310, 13419, 30216] s  tau2_vec=[44, 24, 14, 13419] s  R3_mat=[.014, .382, .407; .028, .006, .007; .014, .007, .006; .333, .956, .912] Ohm  R3_vec=[.382, .006, .007, .956] Ohm  tau3_mat=[1, 44, 5644; 11, 24, 506; 2, 14, 330; 3310, 13419, 30216] s  tau3_vec=[44, 24, 14, 13419] s  R4_mat=[.014, .382, .407; .028, .006, .007; .014, .007, .006; .333, .956, .912] Ohm  R4_vec=[.382, .006, .007, .956] Ohm  tau4_mat=[1, 44, 5644; 11, 24, 506; 2, 14, 330; 3310, 13419, 30216] s  tau4_vec=[44, 24, 14, 13419] s  R5_mat=[.014, .382, .407; .028, .006, .007; .014, .007, .006; .333, .956, .912] Ohm  R5_vec=[.382, .006, .007, .956] Ohm  tau5_mat=[1, 44, 5644; 11, 24, 506; 2, 14, 330; 3310, 13419, 30216] s  tau5_vec=[44, 24, 14, 13419] s  prm_fade=ee.enum.battery.prm_fade.equations  N0=100  dV0=0  dR0=0  dAH=0  dRleak=0  dR1=0  dR2=0  dR3=0  dR4=0  dR5=0  N0vec=[100, 200, 300]  Tfadevec=[298.15, 323.15] K  dV0vec=[0, 0, 0]  dR0vec=[0, 0, 0]  dAHvec=[0, 0, 0]  dRleakvec=[0, 0, 0]  dR1vec=[0, 0, 0]  dR2vec=[0, 0, 0]  dR3vec=[0, 0, 0]  dR4vec=[0, 0, 0]  dR5vec=[0, 0, 0]  dV0mat=[0, 0; 0, 0; 0, 0]  dR0mat=[0, 0; 0, 0; 0, 0]  dAHmat=[0, 0; 0, 0; 0, 0]  dRleakmat=[0, 0; 0, 0; 0, 0]  dR1mat=[0, 0; 0, 0; 0, 0]  dR2mat=[0, 0; 0, 0; 0, 0]  dR3mat=[0, 0; 0, 0; 0, 0]  dR4mat=[0, 0; 0, 0; 0, 0]  dR5mat=[0, 0; 0, 0; 0, 0]  temperature=Battery.TempInit K  i_specify=off  i_priority=None  i=0 A  i_nominal_specify=off  i_nominal_unit=A  i_nominal_value=1  v_specify=off  v_priority=None  v=0 V  v_nominal_specify=off  v_nominal_unit=V  v_nominal_value=1  stateOfCharge_specify=on  stateOfCharge_priority=High  stateOfCharge=(Battery.Capacity_LUT(1) - Battery.Qe_init)/Battery.Capacity_LUT(1)  stateOfCharge_nominal_specify=off  stateOfCharge_nominal_unit=1  stateOfCharge_nominal_value=1  num_cycles_specify=off  num_cycles_priority=High  num_cycles=0  num_cycles_nominal_specify=off  num_cycles_nominal_unit=1  num_cycles_nominal_value=1  thermal_mass=Battery.cell_mass*Battery.cell_Cp_heat J/K  temperature_specify=on  temperature_priority=High  temperature_nominal_specify=off  temperature_nominal_unit=K  temperature_nominal_value=1
      settings: SourceProductName=Simscape Electrical  SourceProductBaseCode=PS  InternalSimscapePortConfiguration="{\"Bottom\":[],\"Left\":[{\"id\":\"p\",\"label\":\"+\",\"type\":\"foundation.electrical.electrical\"},{\"id\":\"soc\",\"label\":\"SOC\",\"type\":\"output\"}],\"Right\":[{\"id\":\"n\",\"label\":\"-\",\"type\":\"foundation.electrical.electrical\"},{\"id\":\"H\",\"label\":\"H\",\"type\":\"foundation.thermal.thermal\"}],\"Top\":[]}"
  Battery_Cell013 : ee_lib/Sources/Battery (Table-Based)  SOC_vec=Battery.SOC_LUT  T_dependence=ee.enum.temperature_dependence.yes  T_vec=Battery.Temperature_LUT K  V0_mat=Battery.Em_LUT V  V0_vec=[3.1, 3.27, 3.31, 3.5] V  R0_mat=Battery.R0_LUT Ohm  R0_vec=[.015, .017, .012, .013] Ohm  AH_vec=Battery.Capacity_LUT hr*A  AH=4.1 hr*A  prm_leak=ee.enum.battery.prm_leak.disabled  Rleak_vec=[8000, 7000, 6000] Ohm  Rleak=7e3 Ohm  prm_dyn=ee.enum.battery.prm_dyn.rc1  R1_mat=Battery.R1_LUT Ohm  R1_vec=[.076, .022, .007, .043] Ohm  tau1_mat=Battery.R1_LUT.*Battery.C1_LUT s  tau1_vec=[148, 110, 27, 22] s  R2_mat=[.014, .382, .407; .028, .006, .007; .014, .007, .006; .333, .956, .912] Ohm  R2_vec=[.382, .006, .007, .956] Ohm  tau2_mat=[1, 44, 5644; 11, 24, 506; 2, 14, 330; 3310, 13419, 30216] s  tau2_vec=[44, 24, 14, 13419] s  R3_mat=[.014, .382, .407; .028, .006, .007; .014, .007, .006; .333, .956, .912] Ohm  R3_vec=[.382, .006, .007, .956] Ohm  tau3_mat=[1, 44, 5644; 11, 24, 506; 2, 14, 330; 3310, 13419, 30216] s  tau3_vec=[44, 24, 14, 13419] s  R4_mat=[.014, .382, .407; .028, .006, .007; .014, .007, .006; .333, .956, .912] Ohm  R4_vec=[.382, .006, .007, .956] Ohm  tau4_mat=[1, 44, 5644; 11, 24, 506; 2, 14, 330; 3310, 13419, 30216] s  tau4_vec=[44, 24, 14, 13419] s  R5_mat=[.014, .382, .407; .028, .006, .007; .014, .007, .006; .333, .956, .912] Ohm  R5_vec=[.382, .006, .007, .956] Ohm  tau5_mat=[1, 44, 5644; 11, 24, 506; 2, 14, 330; 3310, 13419, 30216] s  tau5_vec=[44, 24, 14, 13419] s  prm_fade=ee.enum.battery.prm_fade.equations  N0=100  dV0=0  dR0=0  dAH=0  dRleak=0  dR1=0  dR2=0  dR3=0  dR4=0  dR5=0  N0vec=[100, 200, 300]  Tfadevec=[298.15, 323.15] K  dV0vec=[0, 0, 0]  dR0vec=[0, 0, 0]  dAHvec=[0, 0, 0]  dRleakvec=[0, 0, 0]  dR1vec=[0, 0, 0]  dR2vec=[0, 0, 0]  dR3vec=[0, 0, 0]  dR4vec=[0, 0, 0]  dR5vec=[0, 0, 0]  dV0mat=[0, 0; 0, 0; 0, 0]  dR0mat=[0, 0; 0, 0; 0, 0]  dAHmat=[0, 0; 0, 0; 0, 0]  dRleakmat=[0, 0; 0, 0; 0, 0]  dR1mat=[0, 0; 0, 0; 0, 0]  dR2mat=[0, 0; 0, 0; 0, 0]  dR3mat=[0, 0; 0, 0; 0, 0]  dR4mat=[0, 0; 0, 0; 0, 0]  dR5mat=[0, 0; 0, 0; 0, 0]  temperature=Battery.TempInit K  i_specify=off  i_priority=None  i=0 A  i_nominal_specify=off  i_nominal_unit=A  i_nominal_value=1  v_specify=off  v_priority=None  v=0 V  v_nominal_specify=off  v_nominal_unit=V  v_nominal_value=1  stateOfCharge_specify=on  stateOfCharge_priority=High  stateOfCharge=(Battery.Capacity_LUT(1) - Battery.Qe_init)/Battery.Capacity_LUT(1)  stateOfCharge_nominal_specify=off  stateOfCharge_nominal_unit=1  stateOfCharge_nominal_value=1  num_cycles_specify=off  num_cycles_priority=High  num_cycles=0  num_cycles_nominal_specify=off  num_cycles_nominal_unit=1  num_cycles_nominal_value=1  thermal_mass=Battery.cell_mass*Battery.cell_Cp_heat J/K  temperature_specify=on  temperature_priority=High  temperature_nominal_specify=off  temperature_nominal_unit=K  temperature_nominal_value=1
      settings: SourceProductName=Simscape Electrical  SourceProductBaseCode=PS  InternalSimscapePortConfiguration="{\"Bottom\":[],\"Left\":[{\"id\":\"p\",\"label\":\"+\",\"type\":\"foundation.electrical.electrical\"},{\"id\":\"soc\",\"label\":\"SOC\",\"type\":\"output\"}],\"Right\":[{\"id\":\"n\",\"label\":\"-\",\"type\":\"foundation.electrical.electrical\"},{\"id\":\"H\",\"label\":\"H\",\"type\":\"foundation.thermal.thermal\"}],\"Top\":[]}"
  Battery_Cell014 : ee_lib/Sources/Battery (Table-Based)  SOC_vec=Battery.SOC_LUT  T_dependence=ee.enum.temperature_dependence.yes  T_vec=Battery.Temperature_LUT K  V0_mat=Battery.Em_LUT V  V0_vec=[3.1, 3.27, 3.31, 3.5] V  R0_mat=Battery.R0_LUT Ohm  R0_vec=[.015, .017, .012, .013] Ohm  AH_vec=Battery.Capacity_LUT hr*A  AH=4.1 hr*A  prm_leak=ee.enum.battery.prm_leak.disabled  Rleak_vec=[8000, 7000, 6000] Ohm  Rleak=7e3 Ohm  prm_dyn=ee.enum.battery.prm_dyn.rc1  R1_mat=Battery.R1_LUT Ohm  R1_vec=[.076, .022, .007, .043] Ohm  tau1_mat=Battery.R1_LUT.*Battery.C1_LUT s  tau1_vec=[148, 110, 27, 22] s  R2_mat=[.014, .382, .407; .028, .006, .007; .014, .007, .006; .333, .956, .912] Ohm  R2_vec=[.382, .006, .007, .956] Ohm  tau2_mat=[1, 44, 5644; 11, 24, 506; 2, 14, 330; 3310, 13419, 30216] s  tau2_vec=[44, 24, 14, 13419] s  R3_mat=[.014, .382, .407; .028, .006, .007; .014, .007, .006; .333, .956, .912] Ohm  R3_vec=[.382, .006, .007, .956] Ohm  tau3_mat=[1, 44, 5644; 11, 24, 506; 2, 14, 330; 3310, 13419, 30216] s  tau3_vec=[44, 24, 14, 13419] s  R4_mat=[.014, .382, .407; .028, .006, .007; .014, .007, .006; .333, .956, .912] Ohm  R4_vec=[.382, .006, .007, .956] Ohm  tau4_mat=[1, 44, 5644; 11, 24, 506; 2, 14, 330; 3310, 13419, 30216] s  tau4_vec=[44, 24, 14, 13419] s  R5_mat=[.014, .382, .407; .028, .006, .007; .014, .007, .006; .333, .956, .912] Ohm  R5_vec=[.382, .006, .007, .956] Ohm  tau5_mat=[1, 44, 5644; 11, 24, 506; 2, 14, 330; 3310, 13419, 30216] s  tau5_vec=[44, 24, 14, 13419] s  prm_fade=ee.enum.battery.prm_fade.equations  N0=100  dV0=0  dR0=0  dAH=0  dRleak=0  dR1=0  dR2=0  dR3=0  dR4=0  dR5=0  N0vec=[100, 200, 300]  Tfadevec=[298.15, 323.15] K  dV0vec=[0, 0, 0]  dR0vec=[0, 0, 0]  dAHvec=[0, 0, 0]  dRleakvec=[0, 0, 0]  dR1vec=[0, 0, 0]  dR2vec=[0, 0, 0]  dR3vec=[0, 0, 0]  dR4vec=[0, 0, 0]  dR5vec=[0, 0, 0]  dV0mat=[0, 0; 0, 0; 0, 0]  dR0mat=[0, 0; 0, 0; 0, 0]  dAHmat=[0, 0; 0, 0; 0, 0]  dRleakmat=[0, 0; 0, 0; 0, 0]  dR1mat=[0, 0; 0, 0; 0, 0]  dR2mat=[0, 0; 0, 0; 0, 0]  dR3mat=[0, 0; 0, 0; 0, 0]  dR4mat=[0, 0; 0, 0; 0, 0]  dR5mat=[0, 0; 0, 0; 0, 0]  temperature=Battery.TempInit K  i_specify=off  i_priority=None  i=0 A  i_nominal_specify=off  i_nominal_unit=A  i_nominal_value=1  v_specify=off  v_priority=None  v=0 V  v_nominal_specify=off  v_nominal_unit=V  v_nominal_value=1  stateOfCharge_specify=on  stateOfCharge_priority=High  stateOfCharge=(Battery.Capacity_LUT(1) - Battery.Qe_init)/Battery.Capacity_LUT(1)  stateOfCharge_nominal_specify=off  stateOfCharge_nominal_unit=1  stateOfCharge_nominal_value=1  num_cycles_specify=off  num_cycles_priority=High  num_cycles=0  num_cycles_nominal_specify=off  num_cycles_nominal_unit=1  num_cycles_nominal_value=1  thermal_mass=Battery.cell_mass*Battery.cell_Cp_heat J/K  temperature_specify=on  temperature_priority=High  temperature_nominal_specify=off  temperature_nominal_unit=K  temperature_nominal_value=1
      settings: SourceProductName=Simscape Electrical  SourceProductBaseCode=PS  InternalSimscapePortConfiguration="{\"Bottom\":[],\"Left\":[{\"id\":\"p\",\"label\":\"+\",\"type\":\"foundation.electrical.electrical\"},{\"id\":\"soc\",\"label\":\"SOC\",\"type\":\"output\"}],\"Right\":[{\"id\":\"n\",\"label\":\"-\",\"type\":\"foundation.electrical.electrical\"},{\"id\":\"H\",\"label\":\"H\",\"type\":\"foundation.thermal.thermal\"}],\"Top\":[]}"
  Battery_Cell015 : ee_lib/Sources/Battery (Table-Based)  SOC_vec=Battery.SOC_LUT  T_dependence=ee.enum.temperature_dependence.yes  T_vec=Battery.Temperature_LUT K  V0_mat=Battery.Em_LUT V  V0_vec=[3.1, 3.27, 3.31, 3.5] V  R0_mat=Battery.R0_LUT Ohm  R0_vec=[.015, .017, .012, .013] Ohm  AH_vec=Battery.Capacity_LUT hr*A  AH=4.1 hr*A  prm_leak=ee.enum.battery.prm_leak.disabled  Rleak_vec=[8000, 7000, 6000] Ohm  Rleak=7e3 Ohm  prm_dyn=ee.enum.battery.prm_dyn.rc1  R1_mat=Battery.R1_LUT Ohm  R1_vec=[.076, .022, .007, .043] Ohm  tau1_mat=Battery.R1_LUT.*Battery.C1_LUT s  tau1_vec=[148, 110, 27, 22] s  R2_mat=[.014, .382, .407; .028, .006, .007; .014, .007, .006; .333, .956, .912] Ohm  R2_vec=[.382, .006, .007, .956] Ohm  tau2_mat=[1, 44, 5644; 11, 24, 506; 2, 14, 330; 3310, 13419, 30216] s  tau2_vec=[44, 24, 14, 13419] s  R3_mat=[.014, .382, .407; .028, .006, .007; .014, .007, .006; .333, .956, .912] Ohm  R3_vec=[.382, .006, .007, .956] Ohm  tau3_mat=[1, 44, 5644; 11, 24, 506; 2, 14, 330; 3310, 13419, 30216] s  tau3_vec=[44, 24, 14, 13419] s  R4_mat=[.014, .382, .407; .028, .006, .007; .014, .007, .006; .333, .956, .912] Ohm  R4_vec=[.382, .006, .007, .956] Ohm  tau4_mat=[1, 44, 5644; 11, 24, 506; 2, 14, 330; 3310, 13419, 30216] s  tau4_vec=[44, 24, 14, 13419] s  R5_mat=[.014, .382, .407; .028, .006, .007; .014, .007, .006; .333, .956, .912] Ohm  R5_vec=[.382, .006, .007, .956] Ohm  tau5_mat=[1, 44, 5644; 11, 24, 506; 2, 14, 330; 3310, 13419, 30216] s  tau5_vec=[44, 24, 14, 13419] s  prm_fade=ee.enum.battery.prm_fade.equations  N0=100  dV0=0  dR0=0  dAH=0  dRleak=0  dR1=0  dR2=0  dR3=0  dR4=0  dR5=0  N0vec=[100, 200, 300]  Tfadevec=[298.15, 323.15] K  dV0vec=[0, 0, 0]  dR0vec=[0, 0, 0]  dAHvec=[0, 0, 0]  dRleakvec=[0, 0, 0]  dR1vec=[0, 0, 0]  dR2vec=[0, 0, 0]  dR3vec=[0, 0, 0]  dR4vec=[0, 0, 0]  dR5vec=[0, 0, 0]  dV0mat=[0, 0; 0, 0; 0, 0]  dR0mat=[0, 0; 0, 0; 0, 0]  dAHmat=[0, 0; 0, 0; 0, 0]  dRleakmat=[0, 0; 0, 0; 0, 0]  dR1mat=[0, 0; 0, 0; 0, 0]  dR2mat=[0, 0; 0, 0; 0, 0]  dR3mat=[0, 0; 0, 0; 0, 0]  dR4mat=[0, 0; 0, 0; 0, 0]  dR5mat=[0, 0; 0, 0; 0, 0]  temperature=Battery.TempInit K  i_specify=off  i_priority=None  i=0 A  i_nominal_specify=off  i_nominal_unit=A  i_nominal_value=1  v_specify=off  v_priority=None  v=0 V  v_nominal_specify=off  v_nominal_unit=V  v_nominal_value=1  stateOfCharge_specify=on  stateOfCharge_priority=High  stateOfCharge=(Battery.Capacity_LUT(1) - Battery.Qe_init)/Battery.Capacity_LUT(1)  stateOfCharge_nominal_specify=off  stateOfCharge_nominal_unit=1  stateOfCharge_nominal_value=1  num_cycles_specify=off  num_cycles_priority=High  num_cycles=0  num_cycles_nominal_specify=off  num_cycles_nominal_unit=1  num_cycles_nominal_value=1  thermal_mass=Battery.cell_mass*Battery.cell_Cp_heat J/K  temperature_specify=on  temperature_priority=High  temperature_nominal_specify=off  temperature_nominal_unit=K  temperature_nominal_value=1
      settings: SourceProductName=Simscape Electrical  SourceProductBaseCode=PS  InternalSimscapePortConfiguration="{\"Bottom\":[],\"Left\":[{\"id\":\"p\",\"label\":\"+\",\"type\":\"foundation.electrical.electrical\"},{\"id\":\"soc\",\"label\":\"SOC\",\"type\":\"output\"}],\"Right\":[{\"id\":\"n\",\"label\":\"-\",\"type\":\"foundation.electrical.electrical\"},{\"id\":\"H\",\"label\":\"H\",\"type\":\"foundation.thermal.thermal\"}],\"Top\":[]}"
  Battery_Cell016 : ee_lib/Sources/Battery (Table-Based)  SOC_vec=Battery.SOC_LUT  T_dependence=ee.enum.temperature_dependence.yes  T_vec=Battery.Temperature_LUT K  V0_mat=Battery.Em_LUT V  V0_vec=[3.1, 3.27, 3.31, 3.5] V  R0_mat=Battery.R0_LUT Ohm  R0_vec=[.015, .017, .012, .013] Ohm  AH_vec=Battery.Capacity_LUT hr*A  AH=4.1 hr*A  prm_leak=ee.enum.battery.prm_leak.disabled  Rleak_vec=[8000, 7000, 6000] Ohm  Rleak=7e3 Ohm  prm_dyn=ee.enum.battery.prm_dyn.rc1  R1_mat=Battery.R1_LUT Ohm  R1_vec=[.076, .022, .007, .043] Ohm  tau1_mat=Battery.R1_LUT.*Battery.C1_LUT s  tau1_vec=[148, 110, 27, 22] s  R2_mat=[.014, .382, .407; .028, .006, .007; .014, .007, .006; .333, .956, .912] Ohm  R2_vec=[.382, .006, .007, .956] Ohm  tau2_mat=[1, 44, 5644; 11, 24, 506; 2, 14, 330; 3310, 13419, 30216] s  tau2_vec=[44, 24, 14, 13419] s  R3_mat=[.014, .382, .407; .028, .006, .007; .014, .007, .006; .333, .956, .912] Ohm  R3_vec=[.382, .006, .007, .956] Ohm  tau3_mat=[1, 44, 5644; 11, 24, 506; 2, 14, 330; 3310, 13419, 30216] s  tau3_vec=[44, 24, 14, 13419] s  R4_mat=[.014, .382, .407; .028, .006, .007; .014, .007, .006; .333, .956, .912] Ohm  R4_vec=[.382, .006, .007, .956] Ohm  tau4_mat=[1, 44, 5644; 11, 24, 506; 2, 14, 330; 3310, 13419, 30216] s  tau4_vec=[44, 24, 14, 13419] s  R5_mat=[.014, .382, .407; .028, .006, .007; .014, .007, .006; .333, .956, .912] Ohm  R5_vec=[.382, .006, .007, .956] Ohm  tau5_mat=[1, 44, 5644; 11, 24, 506; 2, 14, 330; 3310, 13419, 30216] s  tau5_vec=[44, 24, 14, 13419] s  prm_fade=ee.enum.battery.prm_fade.equations  N0=100  dV0=0  dR0=0  dAH=0  dRleak=0  dR1=0  dR2=0  dR3=0  dR4=0  dR5=0  N0vec=[100, 200, 300]  Tfadevec=[298.15, 323.15] K  dV0vec=[0, 0, 0]  dR0vec=[0, 0, 0]  dAHvec=[0, 0, 0]  dRleakvec=[0, 0, 0]  dR1vec=[0, 0, 0]  dR2vec=[0, 0, 0]  dR3vec=[0, 0, 0]  dR4vec=[0, 0, 0]  dR5vec=[0, 0, 0]  dV0mat=[0, 0; 0, 0; 0, 0]  dR0mat=[0, 0; 0, 0; 0, 0]  dAHmat=[0, 0; 0, 0; 0, 0]  dRleakmat=[0, 0; 0, 0; 0, 0]  dR1mat=[0, 0; 0, 0; 0, 0]  dR2mat=[0, 0; 0, 0; 0, 0]  dR3mat=[0, 0; 0, 0; 0, 0]  dR4mat=[0, 0; 0, 0; 0, 0]  dR5mat=[0, 0; 0, 0; 0, 0]  temperature=Battery.TempInit K  i_specify=off  i_priority=None  i=0 A  i_nominal_specify=off  i_nominal_unit=A  i_nominal_value=1  v_specify=off  v_priority=None  v=0 V  v_nominal_specify=off  v_nominal_unit=V  v_nominal_value=1  stateOfCharge_specify=on  stateOfCharge_priority=High  stateOfCharge=(Battery.Capacity_LUT(1) - Battery.Qe_init)/Battery.Capacity_LUT(1)  stateOfCharge_nominal_specify=off  stateOfCharge_nominal_unit=1  stateOfCharge_nominal_value=1  num_cycles_specify=off  num_cycles_priority=High  num_cycles=0  num_cycles_nominal_specify=off  num_cycles_nominal_unit=1  num_cycles_nominal_value=1  thermal_mass=Battery.cell_mass*Battery.cell_Cp_heat J/K  temperature_specify=on  temperature_priority=High  temperature_nominal_specify=off  temperature_nominal_unit=K  temperature_nominal_value=1
      settings: SourceProductName=Simscape Electrical  SourceProductBaseCode=PS  InternalSimscapePortConfiguration="{\"Bottom\":[],\"Left\":[{\"id\":\"p\",\"label\":\"+\",\"type\":\"foundation.electrical.electrical\"},{\"id\":\"soc\",\"label\":\"SOC\",\"type\":\"output\"}],\"Right\":[{\"id\":\"n\",\"label\":\"-\",\"type\":\"foundation.electrical.electrical\"},{\"id\":\"H\",\"label\":\"H\",\"type\":\"foundation.thermal.thermal\"}],\"Top\":[]}"
  Compare To Constant{,1..15} (16 alike) : simulink/Logic and Bit Operations/Compare To Constant  relop=<=  const=0.001  OutDataTypeStr=boolean
  Controlled Temperature Source : fl_lib/Thermal/Thermal Sources/Controlled Temperature Source
      settings: SourceProductName=Simscape
  Convective Heat Transfer{,1..15} (16 alike) : fl_lib/Thermal/Thermal Elements/Convective Heat Transfer  area=Battery.cell_area m^2  heat_tr_coeff=Battery.h_conv W/(m^2 * K)  T_specify=off  T_priority=None  T=0 K  T_nominal_specify=off  T_nominal_unit=K  T_nominal_value=1  Q_specify=off  Q_priority=None  Q=0 W  Q_nominal_specify=off  Q_nominal_unit=W  Q_nominal_value=1
  Data Type Conversion{,1..15} (16 alike) : DataTypeConversion  OutDataTypeStr=single
  PS-Simulink Converter{,1..5,14..17,22..25,30..31} (16 alike) : nesl_utility/PS-Simulink Converter  PhysicalDomain=network_engine_domain  SubClassName=ps_output  LeftPortType=input  RightPortType=output  PseudoPeriodic=off  Frequencies=[]  Unit=K  AffineConversion=off
  PS-Simulink Converter{6..13,18..21,26..29} (16 alike) : nesl_utility/PS-Simulink Converter  PhysicalDomain=network_engine_domain  SubClassName=ps_output  LeftPortType=input  RightPortType=output  PseudoPeriodic=off  Frequencies=[]  Unit=1  AffineConversion=off
  Perfect Insulator : fl_lib/Thermal/Thermal Elements/Perfect Insulator  T_specify=off  T_priority=None  T=0 K  T_nominal_specify=off  T_nominal_unit=K  T_nominal_value=1
      settings: SourceProductName=Simscape
  Simulink-PS Converter1 : nesl_utility/Simulink-PS Converter  PhysicalDomain=network_engine_domain  SubClassName=ps_input  LeftPortType=input  RightPortType=output  PseudoPeriodic=off  Frequencies=[]  NoiseDistribution=none  NoiseParameters=[]  Unit=1  AffineConversion=off  FilteringAndDerivatives=provide  SimscapeFilterOrder=1  InputFilterTimeConstant=0.001  UdotUserProvided=0
  Stop Simulation{,1..15} (16 alike) : Stop
  Temperature Sensor{,1..15} (16 alike) : fl_lib/Thermal/Thermal Sensors/Temperature Sensor
  Thermal Reference{,1..16} (17 alike) : fl_lib/Thermal/Thermal Elements/Thermal Reference
  Vector Concatenate : Concatenate  NumInputs=16
  Conn1 : PMIOPort  Side=Right
  Conn2 : PMIOPort  Port=2  Side=Right
  Conn3 : PMIOPort  Port=3  Side=Right
  Conn4 : PMIOPort  Port=4  Side=Right
  Conn5 : PMIOPort  Port=5  Side=Right
  Conn6 : PMIOPort  Port=6  Side=Right
  Conn7 : PMIOPort  Port=7  Side=Right
  Conn8 : PMIOPort  Port=8  Side=Right
  Conn9 : PMIOPort  Port=9  Side=Right
  Conn10 : PMIOPort  Port=10  Side=Right
  Conn11 : PMIOPort  Port=11  Side=Right
  Conn12 : PMIOPort  Port=12  Side=Right
  Conn13 : PMIOPort  Port=13  Side=Right
  Conn14 : PMIOPort  Port=14  Side=Right
  Conn15 : PMIOPort  Port=15  Side=Right
  Conn16 : PMIOPort  Port=16  Side=Right
  Conn17 : PMIOPort  Port=17  Side=Right
  CellTemp : Outport  VectorParamsAs1DForOutWhenUnconnected=off
  wires:
  Compare To Constant14/1 -> Stop Simulation14/1
  PS-Simulink Converter28/1 -> Compare To Constant14/1
  PS-Simulink Converter31/1 -> Data Type Conversion15/1
  Compare To Constant11/1 -> Stop Simulation11/1
  PS-Simulink Converter23/1 -> Data Type Conversion11/1
  Compare To Constant13/1 -> Stop Simulation13/1
  Compare To Constant10/1 -> Stop Simulation10/1
  PS-Simulink Converter24/1 -> Data Type Conversion12/1
  PS-Simulink Converter25/1 -> Data Type Conversion13/1
  PS-Simulink Converter30/1 -> Data Type Conversion14/1
  Data Type Conversion7/1 -> Vector Concatenate/8  "Cell008Temp"
  Data Type Conversion8/1 -> Vector Concatenate/9  "Cell009Temp"
  PS-Simulink Converter14/1 -> Data Type Conversion6/1
  PS-Simulink Converter18/1 -> Compare To Constant6/1
  Compare To Constant6/1 -> Stop Simulation6/1
  PS-Simulink Converter15/1 -> Data Type Conversion7/1
  Compare To Constant9/1 -> Stop Simulation9/1
  PS-Simulink Converter13/1 -> Compare To Constant9/1
  Compare To Constant8/1 -> Stop Simulation8/1
  PS-Simulink Converter16/1 -> Data Type Conversion8/1
  Compare To Constant15/1 -> Stop Simulation15/1
  PS-Simulink Converter27/1 -> Compare To Constant11/1
  PS-Simulink Converter12/1 -> Compare To Constant8/1
  Data Type Conversion3/1 -> Vector Concatenate/4  "Cell004Temp"
  PS-Simulink Converter5/1 -> Data Type Conversion5/1
  Data Type Conversion/1 -> Vector Concatenate/1  "Cell001Temp"
  Compare To Constant/1 -> Stop Simulation/1
  Data Type Conversion1/1 -> Vector Concatenate/2  "Cell002Temp"
  PS-Simulink Converter6/1 -> Compare To Constant/1  "TrueSOC"
  Compare To Constant4/1 -> Stop Simulation4/1
  PS-Simulink Converter21/1 -> Compare To Constant13/1
  PS-Simulink Converter4/1 -> Data Type Conversion4/1
  PS-Simulink Converter1/1 -> Data Type Conversion1/1
  AmbientTemp/1 -> Simulink-PS Converter1/1
  PS-Simulink Converter9/1 -> Compare To Constant3/1
  PS-Simulink Converter2/1 -> Data Type Conversion2/1
  PS-Simulink Converter11/1 -> Compare To Constant5/1
  PS-Simulink Converter19/1 -> Compare To Constant7/1
  PS-Simulink Converter17/1 -> Data Type Conversion9/1
  Vector Concatenate/1 -> CellTemp/1  "CellTemp"
  Compare To Constant1/1 -> Stop Simulation1/1
  Data Type Conversion15/1 -> Vector Concatenate/16  "Cell016Temp"
  Compare To Constant7/1 -> Stop Simulation7/1
  Data Type Conversion14/1 -> Vector Concatenate/15  "Cell015Temp"
  PS-Simulink Converter7/1 -> Compare To Constant1/1
  PS-Simulink Converter10/1 -> Compare To Constant4/1
  PS-Simulink Converter22/1 -> Data Type Conversion10/1
  PS-Simulink Converter8/1 -> Compare To Constant2/1
  Data Type Conversion13/1 -> Vector Concatenate/14  "Cell014Temp"
  Data Type Conversion9/1 -> Vector Concatenate/10  "Cell010Temp"
  Data Type Conversion2/1 -> Vector Concatenate/3  "Cell003Temp"
  Data Type Conversion11/1 -> Vector Concatenate/12  "Cell012Temp"
  Data Type Conversion5/1 -> Vector Concatenate/6  "Cell006Temp"
  Data Type Conversion4/1 -> Vector Concatenate/5  "Cell005Temp"
  Compare To Constant2/1 -> Stop Simulation2/1
  Compare To Constant5/1 -> Stop Simulation5/1
  PS-Simulink Converter29/1 -> Compare To Constant15/1
  PS-Simulink Converter/1 -> Data Type Conversion/1
  Data Type Conversion12/1 -> Vector Concatenate/13  "Cell013Temp"
  Data Type Conversion10/1 -> Vector Concatenate/11  "Cell011Temp"
  PS-Simulink Converter26/1 -> Compare To Constant10/1
  Compare To Constant12/1 -> Stop Simulation12/1
  Data Type Conversion6/1 -> Vector Concatenate/7  "Cell007Temp"
  PS-Simulink Converter20/1 -> Compare To Constant12/1
  PS-Simulink Converter3/1 -> Data Type Conversion3/1
  Compare To Constant3/1 -> Stop Simulation3/1
  connections:
  PS-Simulink Converter28/LConn1 -- Battery_Cell015/LConn2
  Temperature Sensor14/RConn2 -- PS-Simulink Converter30/LConn1
  Thermal Reference11/LConn1 -- Temperature Sensor10/RConn1
  PS-Simulink Converter21/LConn1 -- Battery_Cell014/LConn2
  PS-Simulink Converter26/LConn1 -- Battery_Cell011/LConn2
  Temperature Sensor12/RConn2 -- PS-Simulink Converter24/LConn1
  Thermal Reference13/LConn1 -- Temperature Sensor12/RConn1
  Thermal Reference14/LConn1 -- Temperature Sensor13/RConn1
  Battery_Cell012/RConn2 -- Convective Heat Transfer12/LConn1 -- Temperature Sensor11/LConn1 -- Convective Heat Transfer11/RConn1
  Conn12/RConn1 -- Battery_Cell012/LConn1 -- Battery_Cell011/RConn1
  Battery_Cell013/RConn2 -- Convective Heat Transfer13/LConn1 -- Temperature Sensor12/LConn1 -- Convective Heat Transfer12/RConn1
  PS-Simulink Converter18/LConn1 -- Battery_Cell007/LConn2
  Thermal Reference12/LConn1 -- Temperature Sensor11/RConn1
  Temperature Sensor9/RConn2 -- PS-Simulink Converter17/LConn1
  Thermal Reference7/LConn1 -- Temperature Sensor6/RConn1
  Temperature Sensor7/RConn2 -- PS-Simulink Converter15/LConn1
  PS-Simulink Converter13/LConn1 -- Battery_Cell010/LConn2
  PS-Simulink Converter12/LConn1 -- Battery_Cell009/LConn2
  PS-Simulink Converter19/LConn1 -- Battery_Cell008/LConn2
  Temperature Sensor8/RConn2 -- PS-Simulink Converter16/LConn1
  Battery_Cell007/RConn2 -- Convective Heat Transfer7/LConn1 -- Temperature Sensor6/LConn1 -- Convective Heat Transfer6/RConn1
  Conn10/RConn1 -- Battery_Cell010/LConn1 -- Battery_Cell009/RConn1
  Conn9/RConn1 -- Battery_Cell009/LConn1 -- Battery_Cell008/RConn1
  Conn8/RConn1 -- Battery_Cell008/LConn1 -- Battery_Cell007/RConn1
  PS-Simulink Converter27/LConn1 -- Battery_Cell012/LConn2
  Temperature Sensor6/RConn2 -- PS-Simulink Converter14/LConn1
  Convective Heat Transfer6/LConn1 -- Battery_Cell006/RConn2 -- Convective Heat Transfer5/RConn1 -- Temperature Sensor5/LConn1
  Conn2/RConn1 -- Battery_Cell002/LConn1 -- Battery_Cell001/RConn1
  Conn15/RConn1 -- Battery_Cell014/RConn1 -- Battery_Cell015/LConn1
  Battery_Cell003/RConn2 -- Convective Heat Transfer3/LConn1 -- Temperature Sensor2/LConn1 -- Convective Heat Transfer2/RConn1
  Conn4/RConn1 -- Battery_Cell004/LConn1 -- Battery_Cell003/RConn1
  Temperature Sensor11/RConn2 -- PS-Simulink Converter23/LConn1
  Conn5/RConn1 -- Battery_Cell005/LConn1 -- Battery_Cell004/RConn1
  Conn6/RConn1 -- Battery_Cell006/LConn1 -- Battery_Cell005/RConn1
  PS-Simulink Converter9/LConn1 -- Battery_Cell004/LConn2
  Battery_Cell001/LConn2 -- PS-Simulink Converter6/LConn1
  PS-Simulink Converter8/LConn1 -- Battery_Cell003/LConn2
  Thermal Reference9/LConn1 -- Temperature Sensor8/RConn1
  Temperature Sensor/LConn1 -- Convective Heat Transfer1/LConn1 -- Convective Heat Transfer/RConn1 -- Battery_Cell001/RConn2
  Conn1/RConn1 -- Battery_Cell001/LConn1
  Thermal Reference6/LConn1 -- Temperature Sensor5/RConn1
  Thermal Reference8/LConn1 -- Temperature Sensor7/RConn1
  Temperature Sensor15/RConn2 -- PS-Simulink Converter31/LConn1
  Convective Heat Transfer10/LConn1 -- Temperature Sensor9/LConn1 -- Battery_Cell010/RConn2 -- Convective Heat Transfer9/RConn1
  Temperature Sensor1/RConn2 -- PS-Simulink Converter1/LConn1
  PS-Simulink Converter7/LConn1 -- Battery_Cell002/LConn2
  Simulink-PS Converter1/RConn1 -- Controlled Temperature Source/RConn1
  Conn14/RConn1 -- Battery_Cell014/LConn1 -- Battery_Cell013/RConn1
  Temperature Sensor13/RConn2 -- PS-Simulink Converter25/LConn1
  Conn3/RConn1 -- Battery_Cell003/LConn1 -- Battery_Cell002/RConn1
  Temperature Sensor2/RConn2 -- PS-Simulink Converter2/LConn1
  Convective Heat Transfer/LConn1 -- Controlled Temperature Source/LConn1
  PS-Simulink Converter29/LConn1 -- Battery_Cell016/LConn2
  Thermal Reference1/LConn1 -- Temperature Sensor/RConn1
  Perfect Insulator/LConn1 -- Temperature Sensor15/LConn1 -- Battery_Cell016/RConn2 -- Convective Heat Transfer15/RConn1
  Conn13/RConn1 -- Battery_Cell013/LConn1 -- Battery_Cell012/RConn1
  Temperature Sensor4/RConn2 -- PS-Simulink Converter4/LConn1
  Battery_Cell011/RConn2 -- Convective Heat Transfer11/LConn1 -- Temperature Sensor10/LConn1 -- Convective Heat Transfer10/RConn1
  Temperature Sensor/RConn2 -- PS-Simulink Converter/LConn1
  Thermal Reference4/LConn1 -- Temperature Sensor3/RConn1
  Battery_Cell015/RConn2 -- Convective Heat Transfer15/LConn1 -- Temperature Sensor14/LConn1 -- Convective Heat Transfer14/RConn1
  Battery_Cell004/RConn2 -- Convective Heat Transfer4/LConn1 -- Temperature Sensor3/LConn1 -- Convective Heat Transfer3/RConn1
  Conn7/RConn1 -- Battery_Cell006/RConn1 -- Battery_Cell007/LConn1
  Battery_Cell002/RConn2 -- Convective Heat Transfer2/LConn1 -- Temperature Sensor1/LConn1 -- Convective Heat Transfer1/RConn1
  Conn16/RConn1 -- Battery_Cell016/LConn1 -- Battery_Cell015/RConn1
  Thermal Reference16/LConn1 -- Temperature Sensor15/RConn1
  Temperature Sensor5/RConn2 -- PS-Simulink Converter5/LConn1
  Temperature Sensor3/RConn2 -- PS-Simulink Converter3/LConn1
  Battery_Cell009/RConn2 -- Convective Heat Transfer9/LConn1 -- Temperature Sensor8/LConn1 -- Convective Heat Transfer8/RConn1
  Thermal Reference5/LConn1 -- Temperature Sensor4/RConn1
  PS-Simulink Converter11/LConn1 -- Battery_Cell006/LConn2
  Battery_Cell008/RConn2 -- Convective Heat Transfer8/LConn1 -- Temperature Sensor7/LConn1 -- Convective Heat Transfer7/RConn1
  Battery_Cell016/RConn1 -- Conn17/RConn1
  Thermal Reference15/LConn1 -- Temperature Sensor14/RConn1
  Thermal Reference10/LConn1 -- Temperature Sensor9/RConn1
  Convective Heat Transfer14/LConn1 -- Temperature Sensor13/LConn1 -- Battery_Cell014/RConn2 -- Convective Heat Transfer13/RConn1
  PS-Simulink Converter10/LConn1 -- Battery_Cell005/LConn2
  Battery_Cell005/RConn2 -- Convective Heat Transfer5/LConn1 -- Temperature Sensor4/LConn1 -- Convective Heat Transfer4/RConn1
  Thermal Reference/LConn1 -- Controlled Temperature Source/RConn2
  Temperature Sensor10/RConn2 -- PS-Simulink Converter22/LConn1
  Thermal Reference3/LConn1 -- Temperature Sensor2/RConn1
  Thermal Reference2/LConn1 -- Temperature Sensor1/RConn1
  PS-Simulink Converter20/LConn1 -- Battery_Cell013/LConn2
  Conn11/RConn1 -- Battery_Cell010/RConn1 -- Battery_Cell011/LConn1
